simulink model "Sim_ControladorLQR_Kalman"  (R2025b)
settings: Solver=ode15s  StartTime=0.0  StopTime=10  MaxStep=.0001  RelTol=1e-3
values from neighbouring files (symbols this model uses):
  deg_inicial = 5    [DisenControlKalman.m]
  h = 0.001    [DisenControlKalman.m]
  Kd = dlqr(mG,mH,Q,R)    [DisenControlKalman.m]
  mA = [       0,   1,        0,                 0 ... (first row only)    [Parametros_Proyecto.m]
  mB = [0 ... (first row only)    [Parametros_Proyecto.m]
  mC = eye(4)    [Parametros_Proyecto.m]
  mC_medido = [1, 0, 0, 0 ... (first row only)    [DisenControlKalman.m]
  mD = [0; 0; 0; 0]    [Parametros_Proyecto.m]
  mG = PlantaD.A    [DisenControlKalman.m]
  mH = PlantaD.B    [DisenControlKalman.m]
undefined symbols (not defined in the file or in its folder): Ld
settings Model: Creator=isposzax  LastModifiedBy=alen2

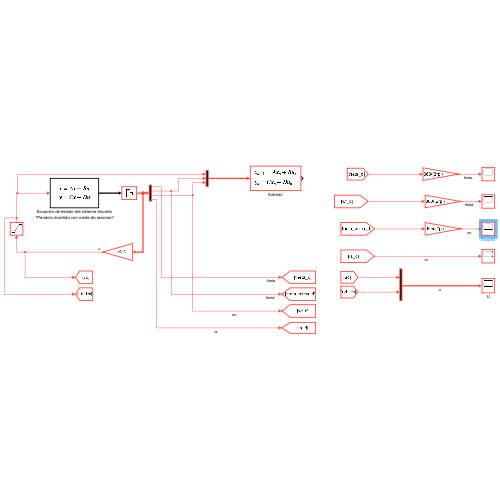
[thumbnail: Simulink's stored preview of the top-level diagram]
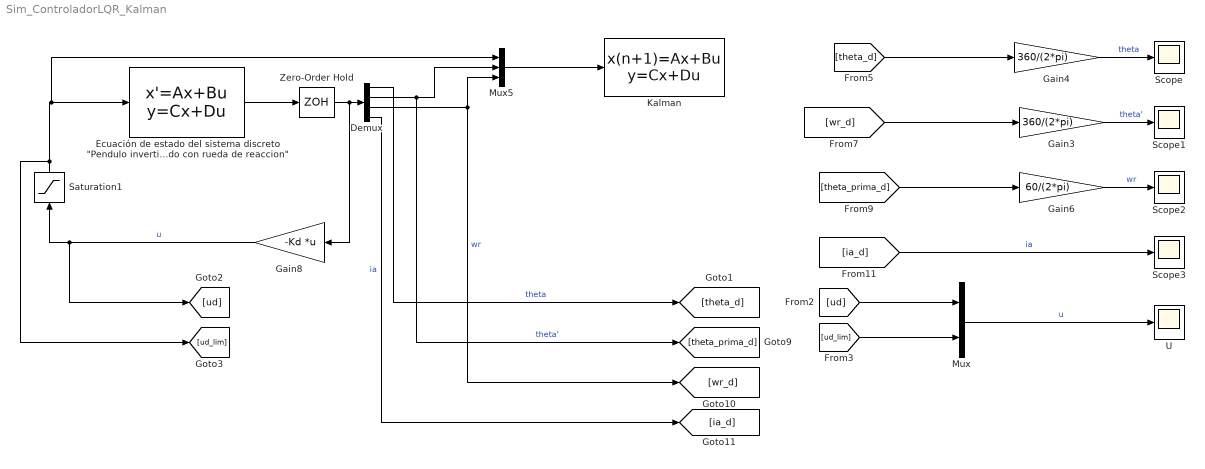
== system Sim_ControladorLQR_Kalman ==
  Demux : Demux
  "Ecuación de estado del sistema discreto \"Pendulo invertido con rueda de reaccion\"" : StateSpace  A=mA  B=mB  C=mC  D=mD  InitialCondition=[deg_inicial*pi/180 0 0 0]
  Gain3 : Gain  Gain=360/(2*pi)
  Gain4 : Gain  Gain=360/(2*pi)
  Gain6 : Gain  Gain=60/(2*pi)
  Gain8 : Gain  Gain=-Kd  Multiplication=Matrix(K*u)
  Kalman : DiscreteStateSpace  A=[mG-Ld*mC_medido]  B=[mH, Ld]  C=eye(size(mG))  D=zeros(4,3)  InitialCondition=[deg_inicial*pi/180; 0; 0; 0]  SampleTime=h
  Mux : Mux  Inputs=2
  Mux5 : Mux  Inputs=3
  Saturation1 : Saturate  UpperLimit=12  LowerLimit=-12
  Scope{,1..3} (4 alike) : Scope
      Scope settings: ActiveDisplayYMinimum=-1.6363472286371787  ActiveDisplayYMaximum=5.7373719142930195
      Scope1 settings: ActiveDisplayYMinimum=-1.2411449420432318E+32  ActiveDisplayYMaximum=1.3790499356035906E+31  DataLoggingVariableName=ScopeData3
      Scope2 settings: ActiveDisplayYMinimum=-2.1914809963512845  ActiveDisplayYMaximum=0.34860772452430977  DataLoggingVariableName=ScopeData4
      Scope3 settings: ActiveDisplayYMinimum=-0.93700965307898132  ActiveDisplayYMaximum=6.18543143791146  DataLoggingVariableName=ScopeData5
  U : Scope
      settings: ActiveDisplayYMinimum=-1.7499722197467678  ActiveDisplayYMaximum=14.941163933086122  DataLoggingVariableName=ScopeData2
  Zero-Order Hold : ZeroOrderHold  SampleTime=h
  wires:
  Gain4/1 -> Scope/1  "theta"
  Gain3/1 -> Scope1/1  "theta'"
  Gain6/1 -> Scope2/1  "wr"
  Gain8/1 -> [ud], Saturation1/1  "u"
  Demux/1 -> [theta_d]  "theta"
  Demux/2 -> [theta_prima_d], Mux5/2  "theta'"
  Demux/3 -> [wr_d], Mux5/3  "wr"
  Demux/4 -> [ia_d]  "ia"
  Mux/1 -> U/1  "u"
  [theta_d] -> Gain4/1
  Saturation1/1 -> Mux5/1, "Ecuación de estado del sistema discreto \"Pendulo invertido con rueda de reaccion\""/1, [ud_lim]
  "Ecuación de estado del sistema discreto \"Pendulo invertido con rueda de reaccion\""/1 -> Zero-Order Hold/1
  Mux5/1 -> Kalman/1
  Zero-Order Hold/1 -> Gain8/1, Demux/1
  [wr_d] -> Gain3/1
  [theta_prima_d] -> Gain6/1
  [ud] -> Mux/1
  [ud_lim] -> Mux/2
  [ia_d] -> Scope3/1  "ia"
